simulink model "IOControls"  (R2019b)
settings: configuration reference "ConfigSet_IOControls_Reference" (kept outside this file)
model workspace (MAT data in the model file):
  SampleTime = 0.05
libraries: IOStateMachinesLib x274, SignalGeneratorsLib x1, simulink x1
(part 7 of 10)

== system IOControls/ForEachVehicle/IOControls/Non-CabControl/CircuitBreakersofEDB/SP4CB ==
  note: States:
      | Tripped
      | Set
  MCBControl : Inport  OutDataTypeStr=Bus: BD_IOControls_In_MCBControl
  Initialise : Inport  Port=2
  Bus Selector : BusSelector  OutputSignals=Value,Mode,InitVal,InternalRequest,Inhibit,TripRequest
  SP4CB-MCB : IOStateMachinesLib/MCB  InitSource=internal  InitState=InitState  OffStateValue=OffStateValue  OnStateValue=OnStateValue
      settings: SourceProductName=IO State Machines
  InputState : Outport  VectorParamsAs1DForOutWhenUnconnected=off
  MCBTripState : Outport  Port=2  VectorParamsAs1DForOutWhenUnconnected=off
  wires:
  SP4CB-MCB/2 -> MCBTripState/1
  Bus Selector/6 -> SP4CB-MCB/7  "<TripRequest>"
  MCBControl/1 -> Bus Selector/1
  Bus Selector/1 -> SP4CB-MCB/1  "<Value>"
  Bus Selector/2 -> SP4CB-MCB/2  "<Mode>"
  Bus Selector/3 -> SP4CB-MCB/3  "<InitVal>"
  Bus Selector/4 -> SP4CB-MCB/5  "<InternalRequest>"
  Bus Selector/5 -> SP4CB-MCB/6  "<Inhibit>"
  SP4CB-MCB/1 -> InputState/1
  Initialise/1 -> SP4CB-MCB/4

== system IOControls/ForEachVehicle/IOControls/Non-CabControl/CircuitBreakersofEDB/SP5CB ==
  note: States:
      | Tripped
      | Set
  MCBControl : Inport  OutDataTypeStr=Bus: BD_IOControls_In_MCBControl
  Initialise : Inport  Port=2
  Bus Selector : BusSelector  OutputSignals=Value,Mode,InitVal,InternalRequest,Inhibit,TripRequest
  SP5CB-MCB : IOStateMachinesLib/MCB  InitSource=internal  InitState=InitState  OffStateValue=OffStateValue  OnStateValue=OnStateValue
      settings: SourceProductName=IO State Machines
  InputState : Outport  VectorParamsAs1DForOutWhenUnconnected=off
  MCBTripState : Outport  Port=2  VectorParamsAs1DForOutWhenUnconnected=off
  wires:
  SP5CB-MCB/2 -> MCBTripState/1
  Bus Selector/6 -> SP5CB-MCB/7  "<TripRequest>"
  MCBControl/1 -> Bus Selector/1
  Bus Selector/1 -> SP5CB-MCB/1  "<Value>"
  Bus Selector/2 -> SP5CB-MCB/2  "<Mode>"
  Bus Selector/3 -> SP5CB-MCB/3  "<InitVal>"
  Bus Selector/4 -> SP5CB-MCB/5  "<InternalRequest>"
  Bus Selector/5 -> SP5CB-MCB/6  "<Inhibit>"
  SP5CB-MCB/1 -> InputState/1
  Initialise/1 -> SP5CB-MCB/4

== system IOControls/ForEachVehicle/IOControls/Non-CabControl/CircuitBreakersofEDB/SP6CB ==
  note: States:
      | Tripped
      | Set
  MCBControl : Inport  OutDataTypeStr=Bus: BD_IOControls_In_MCBControl
  Initialise : Inport  Port=2
  Bus Selector : BusSelector  OutputSignals=Value,Mode,InitVal,InternalRequest,Inhibit,TripRequest
  SP6CB-MCB : IOStateMachinesLib/MCB  InitSource=internal  InitState=InitState  OffStateValue=OffStateValue  OnStateValue=OnStateValue
      settings: SourceProductName=IO State Machines
  InputState : Outport  VectorParamsAs1DForOutWhenUnconnected=off
  MCBTripState : Outport  Port=2  VectorParamsAs1DForOutWhenUnconnected=off
  wires:
  SP6CB-MCB/2 -> MCBTripState/1
  Bus Selector/6 -> SP6CB-MCB/7  "<TripRequest>"
  MCBControl/1 -> Bus Selector/1
  Bus Selector/1 -> SP6CB-MCB/1  "<Value>"
  Bus Selector/2 -> SP6CB-MCB/2  "<Mode>"
  Bus Selector/3 -> SP6CB-MCB/3  "<InitVal>"
  Bus Selector/4 -> SP6CB-MCB/5  "<InternalRequest>"
  Bus Selector/5 -> SP6CB-MCB/6  "<Inhibit>"
  SP6CB-MCB/1 -> InputState/1
  Initialise/1 -> SP6CB-MCB/4

== system IOControls/ForEachVehicle/IOControls/Non-CabControl/CircuitBreakersofEDB/SPCB6 ==
  note: States:
      | Tripped
      | Set
  MCBControl : Inport  OutDataTypeStr=Bus: BD_IOControls_In_MCBControl
  Initialise : Inport  Port=2
  Bus Selector : BusSelector  OutputSignals=Value,Mode,InitVal,InternalRequest,Inhibit,TripRequest
  SPCB6-MCB : IOStateMachinesLib/MCB  InitSource=internal  InitState=InitState  OffStateValue=OffStateValue  OnStateValue=OnStateValue
      settings: SourceProductName=IO State Machines
  InputState : Outport  VectorParamsAs1DForOutWhenUnconnected=off
  MCBTripState : Outport  Port=2  VectorParamsAs1DForOutWhenUnconnected=off
  wires:
  SPCB6-MCB/2 -> MCBTripState/1
  Bus Selector/6 -> SPCB6-MCB/7  "<TripRequest>"
  MCBControl/1 -> Bus Selector/1
  Bus Selector/1 -> SPCB6-MCB/1  "<Value>"
  Bus Selector/2 -> SPCB6-MCB/2  "<Mode>"
  Bus Selector/3 -> SPCB6-MCB/3  "<InitVal>"
  Bus Selector/4 -> SPCB6-MCB/5  "<InternalRequest>"
  Bus Selector/5 -> SPCB6-MCB/6  "<Inhibit>"
  SPCB6-MCB/1 -> InputState/1
  Initialise/1 -> SPCB6-MCB/4

== system IOControls/ForEachVehicle/IOControls/Non-CabControl/CircuitBreakersofEDB/SPCB7 ==
  note: States:
      | Tripped
      | Set
  MCBControl : Inport  OutDataTypeStr=Bus: BD_IOControls_In_MCBControl
  Initialise : Inport  Port=2
  Bus Selector : BusSelector  OutputSignals=Value,Mode,InitVal,InternalRequest,Inhibit,TripRequest
  SPCB7-MCB : IOStateMachinesLib/MCB  InitSource=internal  InitState=InitState  OffStateValue=OffStateValue  OnStateValue=OnStateValue
      settings: SourceProductName=IO State Machines
  InputState : Outport  VectorParamsAs1DForOutWhenUnconnected=off
  MCBTripState : Outport  Port=2  VectorParamsAs1DForOutWhenUnconnected=off
  wires:
  SPCB7-MCB/2 -> MCBTripState/1
  Bus Selector/6 -> SPCB7-MCB/7  "<TripRequest>"
  MCBControl/1 -> Bus Selector/1
  Bus Selector/1 -> SPCB7-MCB/1  "<Value>"
  Bus Selector/2 -> SPCB7-MCB/2  "<Mode>"
  Bus Selector/3 -> SPCB7-MCB/3  "<InitVal>"
  Bus Selector/4 -> SPCB7-MCB/5  "<InternalRequest>"
  Bus Selector/5 -> SPCB7-MCB/6  "<Inhibit>"
  SPCB7-MCB/1 -> InputState/1
  Initialise/1 -> SPCB7-MCB/4

== system IOControls/ForEachVehicle/IOControls/Non-CabControl/CircuitBreakersofEDB/SPCB8 ==
  note: States:
      | Tripped
      | Set
  MCBControl : Inport  OutDataTypeStr=Bus: BD_IOControls_In_MCBControl
  Initialise : Inport  Port=2
  Bus Selector : BusSelector  OutputSignals=Value,Mode,InitVal,InternalRequest,Inhibit,TripRequest
  SPCB8-MCB : IOStateMachinesLib/MCB  InitSource=internal  InitState=InitState  OffStateValue=OffStateValue  OnStateValue=OnStateValue
      settings: SourceProductName=IO State Machines
  InputState : Outport  VectorParamsAs1DForOutWhenUnconnected=off
  MCBTripState : Outport  Port=2  VectorParamsAs1DForOutWhenUnconnected=off
  wires:
  SPCB8-MCB/2 -> MCBTripState/1
  Bus Selector/6 -> SPCB8-MCB/7  "<TripRequest>"
  MCBControl/1 -> Bus Selector/1
  Bus Selector/1 -> SPCB8-MCB/1  "<Value>"
  Bus Selector/2 -> SPCB8-MCB/2  "<Mode>"
  Bus Selector/3 -> SPCB8-MCB/3  "<InitVal>"
  Bus Selector/4 -> SPCB8-MCB/5  "<InternalRequest>"
  Bus Selector/5 -> SPCB8-MCB/6  "<Inhibit>"
  SPCB8-MCB/1 -> InputState/1
  Initialise/1 -> SPCB8-MCB/4

== system IOControls/ForEachVehicle/IOControls/Non-CabControl/CircuitBreakersofEDB/SPPB ==
  note: States:
      | Off
      | On
  InputControl : Inport  OutDataTypeStr=Bus: BD_IOControls_In_InputControl
  Initialise : Inport  Port=2
  Bus Selector : BusSelector  OutputSignals=Value,Mode,InitVal,InternalRequest,Inhibit
  SPPB-Momentary : IOStateMachinesLib/Momentary  InitSource=internal  InitState=InitState
      settings: SourceProductName=IO State Machines
  InputState : Outport  VectorParamsAs1DForOutWhenUnconnected=off
  wires:
  Initialise/1 -> SPPB-Momentary/4
  SPPB-Momentary/1 -> InputState/1
  Bus Selector/5 -> SPPB-Momentary/6  "<Inhibit>"
  Bus Selector/4 -> SPPB-Momentary/5  "<InternalRequest>"
  Bus Selector/3 -> SPPB-Momentary/3  "<InitVal>"
  Bus Selector/2 -> SPPB-Momentary/2  "<Mode>"
  Bus Selector/1 -> SPPB-Momentary/1  "<Value>"
  InputControl/1 -> Bus Selector/1

== system IOControls/ForEachVehicle/IOControls/Non-CabControl/CircuitBreakersofEDB/SPSW ==
  note: States:
      | Normal
      | Cutout
  InputControl : Inport  OutDataTypeStr=Bus: BD_IOControls_In_InputControl
  Initialise : Inport  Port=2
  Bus Selector : BusSelector  OutputSignals=Value,Mode,InitVal,InternalRequest,Inhibit
  SPSW-Toggle : IOStateMachinesLib/Toggle  InitSource=internal  InitState=InitState  OffStateValue=OffStateValue  OnStateValue=OnStateValue
      settings: SourceProductName=IO State Machines
  InputState : Outport  VectorParamsAs1DForOutWhenUnconnected=off
  wires:
  Initialise/1 -> SPSW-Toggle/4
  SPSW-Toggle/1 -> InputState/1
  Bus Selector/5 -> SPSW-Toggle/6  "<Inhibit>"
  Bus Selector/4 -> SPSW-Toggle/5  "<InternalRequest>"
  Bus Selector/3 -> SPSW-Toggle/3  "<InitVal>"
  Bus Selector/2 -> SPSW-Toggle/2  "<Mode>"
  Bus Selector/1 -> SPSW-Toggle/1  "<Value>"
  InputControl/1 -> Bus Selector/1

== system IOControls/ForEachVehicle/IOControls/Non-CabControl/CircuitBreakersofEDB/SSCB ==
  note: States:
      | Tripped
      | Set
  MCBControl : Inport  OutDataTypeStr=Bus: BD_IOControls_In_MCBControl
  Initialise : Inport  Port=2
  Bus Selector : BusSelector  OutputSignals=Value,Mode,InitVal,InternalRequest,Inhibit,TripRequest
  SSCB-MCB : IOStateMachinesLib/MCB  InitSource=internal  InitState=InitState  OffStateValue=OffStateValue  OnStateValue=OnStateValue
      settings: SourceProductName=IO State Machines
  InputState : Outport  VectorParamsAs1DForOutWhenUnconnected=off
  MCBTripState : Outport  Port=2  VectorParamsAs1DForOutWhenUnconnected=off
  wires:
  SSCB-MCB/2 -> MCBTripState/1
  Bus Selector/6 -> SSCB-MCB/7  "<TripRequest>"
  MCBControl/1 -> Bus Selector/1
  Bus Selector/1 -> SSCB-MCB/1  "<Value>"
  Bus Selector/2 -> SSCB-MCB/2  "<Mode>"
  Bus Selector/3 -> SSCB-MCB/3  "<InitVal>"
  Bus Selector/4 -> SSCB-MCB/5  "<InternalRequest>"
  Bus Selector/5 -> SSCB-MCB/6  "<Inhibit>"
  SSCB-MCB/1 -> InputState/1
  Initialise/1 -> SSCB-MCB/4

== system IOControls/ForEachVehicle/IOControls/Non-CabControl/CircuitBreakersofEDB/SSICB ==
  note: States:
      | Tripped
      | Set
  MCBControl : Inport  OutDataTypeStr=Bus: BD_IOControls_In_MCBControl
  Initialise : Inport  Port=2
  Bus Selector : BusSelector  OutputSignals=Value,Mode,InitVal,InternalRequest,Inhibit,TripRequest
  SSICB-MCB : IOStateMachinesLib/MCB  InitSource=internal  InitState=InitState  OffStateValue=OffStateValue  OnStateValue=OnStateValue
      settings: SourceProductName=IO State Machines
  InputState : Outport  VectorParamsAs1DForOutWhenUnconnected=off
  MCBTripState : Outport  Port=2  VectorParamsAs1DForOutWhenUnconnected=off
  wires:
  SSICB-MCB/2 -> MCBTripState/1
  Bus Selector/6 -> SSICB-MCB/7  "<TripRequest>"
  MCBControl/1 -> Bus Selector/1
  Bus Selector/1 -> SSICB-MCB/1  "<Value>"
  Bus Selector/2 -> SSICB-MCB/2  "<Mode>"
  Bus Selector/3 -> SSICB-MCB/3  "<InitVal>"
  Bus Selector/4 -> SSICB-MCB/5  "<InternalRequest>"
  Bus Selector/5 -> SSICB-MCB/6  "<Inhibit>"
  SSICB-MCB/1 -> InputState/1
  Initialise/1 -> SSICB-MCB/4

== system IOControls/ForEachVehicle/IOControls/Non-CabControl/CircuitBreakersofEDB/TBCCB1 ==
  note: States:
      | Tripped
      | Set
  MCBControl : Inport  OutDataTypeStr=Bus: BD_IOControls_In_MCBControl
  Initialise : Inport  Port=2
  Bus Selector : BusSelector  OutputSignals=Value,Mode,InitVal,InternalRequest,Inhibit,TripRequest
  TBCCB1-MCB : IOStateMachinesLib/MCB  InitSource=internal  InitState=InitState  OffStateValue=OffStateValue  OnStateValue=OnStateValue
      settings: SourceProductName=IO State Machines
  InputState : Outport  VectorParamsAs1DForOutWhenUnconnected=off
  MCBTripState : Outport  Port=2  VectorParamsAs1DForOutWhenUnconnected=off
  wires:
  TBCCB1-MCB/2 -> MCBTripState/1
  Bus Selector/6 -> TBCCB1-MCB/7  "<TripRequest>"
  MCBControl/1 -> Bus Selector/1
  Bus Selector/1 -> TBCCB1-MCB/1  "<Value>"
  Bus Selector/2 -> TBCCB1-MCB/2  "<Mode>"
  Bus Selector/3 -> TBCCB1-MCB/3  "<InitVal>"
  Bus Selector/4 -> TBCCB1-MCB/5  "<InternalRequest>"
  Bus Selector/5 -> TBCCB1-MCB/6  "<Inhibit>"
  TBCCB1-MCB/1 -> InputState/1
  Initialise/1 -> TBCCB1-MCB/4

== system IOControls/ForEachVehicle/IOControls/Non-CabControl/CircuitBreakersofEDB/TBCCB2 ==
  note: States:
      | Tripped
      | Set
  MCBControl : Inport  OutDataTypeStr=Bus: BD_IOControls_In_MCBControl
  Initialise : Inport  Port=2
  Bus Selector : BusSelector  OutputSignals=Value,Mode,InitVal,InternalRequest,Inhibit,TripRequest
  TBCCB2-MCB : IOStateMachinesLib/MCB  InitSource=internal  InitState=InitState  OffStateValue=OffStateValue  OnStateValue=OnStateValue
      settings: SourceProductName=IO State Machines
  InputState : Outport  VectorParamsAs1DForOutWhenUnconnected=off
  MCBTripState : Outport  Port=2  VectorParamsAs1DForOutWhenUnconnected=off
  wires:
  TBCCB2-MCB/2 -> MCBTripState/1
  Bus Selector/6 -> TBCCB2-MCB/7  "<TripRequest>"
  MCBControl/1 -> Bus Selector/1
  Bus Selector/1 -> TBCCB2-MCB/1  "<Value>"
  Bus Selector/2 -> TBCCB2-MCB/2  "<Mode>"
  Bus Selector/3 -> TBCCB2-MCB/3  "<InitVal>"
  Bus Selector/4 -> TBCCB2-MCB/5  "<InternalRequest>"
  Bus Selector/5 -> TBCCB2-MCB/6  "<Inhibit>"
  TBCCB2-MCB/1 -> InputState/1
  Initialise/1 -> TBCCB2-MCB/4

== system IOControls/ForEachVehicle/IOControls/Non-CabControl/CircuitBreakersofEDB/TBNCB ==
  note: States:
      | Tripped
      | Set
  MCBControl : Inport  OutDataTypeStr=Bus: BD_IOControls_In_MCBControl
  Initialise : Inport  Port=2
  Bus Selector : BusSelector  OutputSignals=Value,Mode,InitVal,InternalRequest,Inhibit,TripRequest
  TBNCB-MCB : IOStateMachinesLib/MCB  InitSource=internal  InitState=InitState  OffStateValue=OffStateValue  OnStateValue=OnStateValue
      settings: SourceProductName=IO State Machines
  InputState : Outport  VectorParamsAs1DForOutWhenUnconnected=off
  MCBTripState : Outport  Port=2  VectorParamsAs1DForOutWhenUnconnected=off
  wires:
  TBNCB-MCB/2 -> MCBTripState/1
  Bus Selector/6 -> TBNCB-MCB/7  "<TripRequest>"
  MCBControl/1 -> Bus Selector/1
  Bus Selector/1 -> TBNCB-MCB/1  "<Value>"
  Bus Selector/2 -> TBNCB-MCB/2  "<Mode>"
  Bus Selector/3 -> TBNCB-MCB/3  "<InitVal>"
  Bus Selector/4 -> TBNCB-MCB/5  "<InternalRequest>"
  Bus Selector/5 -> TBNCB-MCB/6  "<Inhibit>"
  TBNCB-MCB/1 -> InputState/1
  Initialise/1 -> TBNCB-MCB/4

== system IOControls/ForEachVehicle/IOControls/Non-CabControl/CircuitBreakersofEDB/TDICB ==
  note: States:
      | Tripped
      | Set
  MCBControl : Inport  OutDataTypeStr=Bus: BD_IOControls_In_MCBControl
  Initialise : Inport  Port=2
  Bus Selector : BusSelector  OutputSignals=Value,Mode,InitVal,InternalRequest,Inhibit,TripRequest
  TDICB-MCB : IOStateMachinesLib/MCB  InitSource=internal  InitState=InitState  OffStateValue=OffStateValue  OnStateValue=OnStateValue
      settings: SourceProductName=IO State Machines
  InputState : Outport  VectorParamsAs1DForOutWhenUnconnected=off
  MCBTripState : Outport  Port=2  VectorParamsAs1DForOutWhenUnconnected=off
  wires:
  TDICB-MCB/2 -> MCBTripState/1
  Bus Selector/6 -> TDICB-MCB/7  "<TripRequest>"
  MCBControl/1 -> Bus Selector/1
  Bus Selector/1 -> TDICB-MCB/1  "<Value>"
  Bus Selector/2 -> TDICB-MCB/2  "<Mode>"
  Bus Selector/3 -> TDICB-MCB/3  "<InitVal>"
  Bus Selector/4 -> TDICB-MCB/5  "<InternalRequest>"
  Bus Selector/5 -> TDICB-MCB/6  "<Inhibit>"
  TDICB-MCB/1 -> InputState/1
  Initialise/1 -> TDICB-MCB/4

== system IOControls/ForEachVehicle/IOControls/Non-CabControl/CircuitBreakersofEDB/TERCB1 ==
  note: States:
      | Tripped
      | Set
  MCBControl : Inport  OutDataTypeStr=Bus: BD_IOControls_In_MCBControl
  Initialise : Inport  Port=2
  Bus Selector : BusSelector  OutputSignals=Value,Mode,InitVal,InternalRequest,Inhibit,TripRequest
  TERCB1-MCB : IOStateMachinesLib/MCB  InitSource=internal  InitState=InitState  OffStateValue=OffStateValue  OnStateValue=OnStateValue
      settings: SourceProductName=IO State Machines
  InputState : Outport  VectorParamsAs1DForOutWhenUnconnected=off
  MCBTripState : Outport  Port=2  VectorParamsAs1DForOutWhenUnconnected=off
  wires:
  TERCB1-MCB/2 -> MCBTripState/1
  Bus Selector/6 -> TERCB1-MCB/7  "<TripRequest>"
  MCBControl/1 -> Bus Selector/1
  Bus Selector/1 -> TERCB1-MCB/1  "<Value>"
  Bus Selector/2 -> TERCB1-MCB/2  "<Mode>"
  Bus Selector/3 -> TERCB1-MCB/3  "<InitVal>"
  Bus Selector/4 -> TERCB1-MCB/5  "<InternalRequest>"
  Bus Selector/5 -> TERCB1-MCB/6  "<Inhibit>"
  TERCB1-MCB/1 -> InputState/1
  Initialise/1 -> TERCB1-MCB/4

== system IOControls/ForEachVehicle/IOControls/Non-CabControl/CircuitBreakersofEDB/TERCB2 ==
  note: States:
      | Tripped
      | Set
  MCBControl : Inport  OutDataTypeStr=Bus: BD_IOControls_In_MCBControl
  Initialise : Inport  Port=2
  Bus Selector : BusSelector  OutputSignals=Value,Mode,InitVal,InternalRequest,Inhibit,TripRequest
  TERCB2-MCB : IOStateMachinesLib/MCB  InitSource=internal  InitState=InitState  OffStateValue=OffStateValue  OnStateValue=OnStateValue
      settings: SourceProductName=IO State Machines
  InputState : Outport  VectorParamsAs1DForOutWhenUnconnected=off
  MCBTripState : Outport  Port=2  VectorParamsAs1DForOutWhenUnconnected=off
  wires:
  TERCB2-MCB/2 -> MCBTripState/1
  Bus Selector/6 -> TERCB2-MCB/7  "<TripRequest>"
  MCBControl/1 -> Bus Selector/1
  Bus Selector/1 -> TERCB2-MCB/1  "<Value>"
  Bus Selector/2 -> TERCB2-MCB/2  "<Mode>"
  Bus Selector/3 -> TERCB2-MCB/3  "<InitVal>"
  Bus Selector/4 -> TERCB2-MCB/5  "<InternalRequest>"
  Bus Selector/5 -> TERCB2-MCB/6  "<Inhibit>"
  TERCB2-MCB/1 -> InputState/1
  Initialise/1 -> TERCB2-MCB/4

== system IOControls/ForEachVehicle/IOControls/Non-CabControl/CircuitBreakersofEDB/TLLCB ==
  note: States:
      | Tripped
      | Set
  MCBControl : Inport  OutDataTypeStr=Bus: BD_IOControls_In_MCBControl
  Initialise : Inport  Port=2
  Bus Selector : BusSelector  OutputSignals=Value,Mode,InitVal,InternalRequest,Inhibit,TripRequest
  TLLCB-MCB : IOStateMachinesLib/MCB  InitSource=internal  InitState=InitState  OffStateValue=OffStateValue  OnStateValue=OnStateValue
      settings: SourceProductName=IO State Machines
  InputState : Outport  VectorParamsAs1DForOutWhenUnconnected=off
  MCBTripState : Outport  Port=2  VectorParamsAs1DForOutWhenUnconnected=off
  wires:
  TLLCB-MCB/2 -> MCBTripState/1
  Bus Selector/6 -> TLLCB-MCB/7  "<TripRequest>"
  MCBControl/1 -> Bus Selector/1
  Bus Selector/1 -> TLLCB-MCB/1  "<Value>"
  Bus Selector/2 -> TLLCB-MCB/2  "<Mode>"
  Bus Selector/3 -> TLLCB-MCB/3  "<InitVal>"
  Bus Selector/4 -> TLLCB-MCB/5  "<InternalRequest>"
  Bus Selector/5 -> TLLCB-MCB/6  "<Inhibit>"
  TLLCB-MCB/1 -> InputState/1
  Initialise/1 -> TLLCB-MCB/4

== system IOControls/ForEachVehicle/IOControls/Non-CabControl/CircuitBreakersofEDB/TLRCB ==
  note: States:
      | Tripped
      | Set
  MCBControl : Inport  OutDataTypeStr=Bus: BD_IOControls_In_MCBControl
  Initialise : Inport  Port=2
  Bus Selector : BusSelector  OutputSignals=Value,Mode,InitVal,InternalRequest,Inhibit,TripRequest
  TLRCB-MCB : IOStateMachinesLib/MCB  InitSource=internal  InitState=InitState  OffStateValue=OffStateValue  OnStateValue=OnStateValue
      settings: SourceProductName=IO State Machines
  InputState : Outport  VectorParamsAs1DForOutWhenUnconnected=off
  MCBTripState : Outport  Port=2  VectorParamsAs1DForOutWhenUnconnected=off
  wires:
  TLRCB-MCB/2 -> MCBTripState/1
  Bus Selector/6 -> TLRCB-MCB/7  "<TripRequest>"
  MCBControl/1 -> Bus Selector/1
  Bus Selector/1 -> TLRCB-MCB/1  "<Value>"
  Bus Selector/2 -> TLRCB-MCB/2  "<Mode>"
  Bus Selector/3 -> TLRCB-MCB/3  "<InitVal>"
  Bus Selector/4 -> TLRCB-MCB/5  "<InternalRequest>"
  Bus Selector/5 -> TLRCB-MCB/6  "<Inhibit>"
  TLRCB-MCB/1 -> InputState/1
  Initialise/1 -> TLRCB-MCB/4

== system IOControls/ForEachVehicle/IOControls/Non-CabControl/CircuitBreakersofEDB/TRIVCB ==
  note: States:
      | Tripped
      | Set
  MCBControl : Inport  OutDataTypeStr=Bus: BD_IOControls_In_MCBControl
  Initialise : Inport  Port=2
  Bus Selector : BusSelector  OutputSignals=Value,Mode,InitVal,InternalRequest,Inhibit,TripRequest
  TRIVCB-MCB : IOStateMachinesLib/MCB  InitSource=internal  InitState=InitState  OffStateValue=OffStateValue  OnStateValue=OnStateValue
      settings: SourceProductName=IO State Machines
  InputState : Outport  VectorParamsAs1DForOutWhenUnconnected=off
  MCBTripState : Outport  Port=2  VectorParamsAs1DForOutWhenUnconnected=off
  wires:
  TRIVCB-MCB/2 -> MCBTripState/1
  Bus Selector/6 -> TRIVCB-MCB/7  "<TripRequest>"
  MCBControl/1 -> Bus Selector/1
  Bus Selector/1 -> TRIVCB-MCB/1  "<Value>"
  Bus Selector/2 -> TRIVCB-MCB/2  "<Mode>"
  Bus Selector/3 -> TRIVCB-MCB/3  "<InitVal>"
  Bus Selector/4 -> TRIVCB-MCB/5  "<InternalRequest>"
  Bus Selector/5 -> TRIVCB-MCB/6  "<Inhibit>"
  TRIVCB-MCB/1 -> InputState/1
  Initialise/1 -> TRIVCB-MCB/4

== system IOControls/ForEachVehicle/IOControls/Non-CabControl/CircuitBreakersofEDB/TVDUCB ==
  note: States:
      | Tripped
      | Set
  MCBControl : Inport  OutDataTypeStr=Bus: BD_IOControls_In_MCBControl
  Initialise : Inport  Port=2
  Bus Selector : BusSelector  OutputSignals=Value,Mode,InitVal,InternalRequest,Inhibit,TripRequest
  TVDUCB-MCB : IOStateMachinesLib/MCB  InitSource=internal  InitState=InitState  OffStateValue=OffStateValue  OnStateValue=OnStateValue
      settings: SourceProductName=IO State Machines
  InputState : Outport  VectorParamsAs1DForOutWhenUnconnected=off
  MCBTripState : Outport  Port=2  VectorParamsAs1DForOutWhenUnconnected=off
  wires:
  TVDUCB-MCB/2 -> MCBTripState/1
  Bus Selector/6 -> TVDUCB-MCB/7  "<TripRequest>"
  MCBControl/1 -> Bus Selector/1
  Bus Selector/1 -> TVDUCB-MCB/1  "<Value>"
  Bus Selector/2 -> TVDUCB-MCB/2  "<Mode>"
  Bus Selector/3 -> TVDUCB-MCB/3  "<InitVal>"
  Bus Selector/4 -> TVDUCB-MCB/5  "<InternalRequest>"
  Bus Selector/5 -> TVDUCB-MCB/6  "<Inhibit>"
  TVDUCB-MCB/1 -> InputState/1
  Initialise/1 -> TVDUCB-MCB/4

== system IOControls/ForEachVehicle/IOControls/Non-CabControl/CircuitBreakersofEDB/TWVCB ==
  note: States:
      | Tripped
      | Set
  MCBControl : Inport  OutDataTypeStr=Bus: BD_IOControls_In_MCBControl
  Initialise : Inport  Port=2
  Bus Selector : BusSelector  OutputSignals=Value,Mode,InitVal,InternalRequest,Inhibit,TripRequest
  TWVCB-MCB : IOStateMachinesLib/MCB  InitSource=internal  InitState=InitState  OffStateValue=OffStateValue  OnStateValue=OnStateValue
      settings: SourceProductName=IO State Machines
  InputState : Outport  VectorParamsAs1DForOutWhenUnconnected=off
  MCBTripState : Outport  Port=2  VectorParamsAs1DForOutWhenUnconnected=off
  wires:
  TWVCB-MCB/2 -> MCBTripState/1
  Bus Selector/6 -> TWVCB-MCB/7  "<TripRequest>"
  MCBControl/1 -> Bus Selector/1
  Bus Selector/1 -> TWVCB-MCB/1  "<Value>"
  Bus Selector/2 -> TWVCB-MCB/2  "<Mode>"
  Bus Selector/3 -> TWVCB-MCB/3  "<InitVal>"
  Bus Selector/4 -> TWVCB-MCB/5  "<InternalRequest>"
  Bus Selector/5 -> TWVCB-MCB/6  "<Inhibit>"
  TWVCB-MCB/1 -> InputState/1
  Initialise/1 -> TWVCB-MCB/4

== system IOControls/ForEachVehicle/IOControls/Non-CabControl/CircuitBreakersofEDB/VCBCB ==
  note: States:
      | Tripped
      | Set
  MCBControl : Inport  OutDataTypeStr=Bus: BD_IOControls_In_MCBControl
  Initialise : Inport  Port=2
  Bus Selector : BusSelector  OutputSignals=Value,Mode,InitVal,InternalRequest,Inhibit,TripRequest
  VCBCB-MCB : IOStateMachinesLib/MCB  InitSource=internal  InitState=InitState  OffStateValue=OffStateValue  OnStateValue=OnStateValue
      settings: SourceProductName=IO State Machines
  InputState : Outport  VectorParamsAs1DForOutWhenUnconnected=off
  MCBTripState : Outport  Port=2  VectorParamsAs1DForOutWhenUnconnected=off
  wires:
  VCBCB-MCB/2 -> MCBTripState/1
  Bus Selector/6 -> VCBCB-MCB/7  "<TripRequest>"
  MCBControl/1 -> Bus Selector/1
  Bus Selector/1 -> VCBCB-MCB/1  "<Value>"
  Bus Selector/2 -> VCBCB-MCB/2  "<Mode>"
  Bus Selector/3 -> VCBCB-MCB/3  "<InitVal>"
  Bus Selector/4 -> VCBCB-MCB/5  "<InternalRequest>"
  Bus Selector/5 -> VCBCB-MCB/6  "<Inhibit>"
  VCBCB-MCB/1 -> InputState/1
  Initialise/1 -> VCBCB-MCB/4

== system IOControls/ForEachVehicle/IOControls/Non-CabControl/CircuitBreakersofEDB/VCBCCB ==
  note: States:
      | Tripped
      | Set
  MCBControl : Inport  OutDataTypeStr=Bus: BD_IOControls_In_MCBControl
  Initialise : Inport  Port=2
  Bus Selector : BusSelector  OutputSignals=Value,Mode,InitVal,InternalRequest,Inhibit,TripRequest
  VCBCCB-MCB : IOStateMachinesLib/MCB  InitSource=internal  InitState=InitState  OffStateValue=OffStateValue  OnStateValue=OnStateValue
      settings: SourceProductName=IO State Machines
  InputState : Outport  VectorParamsAs1DForOutWhenUnconnected=off
  MCBTripState : Outport  Port=2  VectorParamsAs1DForOutWhenUnconnected=off
  wires:
  VCBCCB-MCB/2 -> MCBTripState/1
  Bus Selector/6 -> VCBCCB-MCB/7  "<TripRequest>"
  MCBControl/1 -> Bus Selector/1
  Bus Selector/1 -> VCBCCB-MCB/1  "<Value>"
  Bus Selector/2 -> VCBCCB-MCB/2  "<Mode>"
  Bus Selector/3 -> VCBCCB-MCB/3  "<InitVal>"
  Bus Selector/4 -> VCBCCB-MCB/5  "<InternalRequest>"
  Bus Selector/5 -> VCBCCB-MCB/6  "<Inhibit>"
  VCBCCB-MCB/1 -> InputState/1
  Initialise/1 -> VCBCCB-MCB/4

== system IOControls/ForEachVehicle/IOControls/Non-CabControl/CircuitBreakersofEDB/VCCBOrUCCB ==
  note: States:
      | Tripped
      | Set
  MCBControl : Inport  OutDataTypeStr=Bus: BD_IOControls_In_MCBControl
  Initialise : Inport  Port=2
  Bus Selector : BusSelector  OutputSignals=Value,Mode,InitVal,InternalRequest,Inhibit,TripRequest
  VCCBOrUCCB-MCB : IOStateMachinesLib/MCB  InitSource=internal  InitState=InitState  OffStateValue=OffStateValue  OnStateValue=OnStateValue
      settings: SourceProductName=IO State Machines
  InputState : Outport  VectorParamsAs1DForOutWhenUnconnected=off
  MCBTripState : Outport  Port=2  VectorParamsAs1DForOutWhenUnconnected=off
  wires:
  VCCBOrUCCB-MCB/2 -> MCBTripState/1
  Bus Selector/6 -> VCCBOrUCCB-MCB/7  "<TripRequest>"
  MCBControl/1 -> Bus Selector/1
  Bus Selector/1 -> VCCBOrUCCB-MCB/1  "<Value>"
  Bus Selector/2 -> VCCBOrUCCB-MCB/2  "<Mode>"
  Bus Selector/3 -> VCCBOrUCCB-MCB/3  "<InitVal>"
  Bus Selector/4 -> VCCBOrUCCB-MCB/5  "<InternalRequest>"
  Bus Selector/5 -> VCCBOrUCCB-MCB/6  "<Inhibit>"
  VCCBOrUCCB-MCB/1 -> InputState/1
  Initialise/1 -> VCCBOrUCCB-MCB/4

== system IOControls/ForEachVehicle/IOControls/Non-CabControl/CircuitBreakersofEDB/VIO1CB ==
  note: States:
      | Tripped
      | Set
  MCBControl : Inport  OutDataTypeStr=Bus: BD_IOControls_In_MCBControl
  Initialise : Inport  Port=2
  Bus Selector : BusSelector  OutputSignals=Value,Mode,InitVal,InternalRequest,Inhibit,TripRequest
  VIO1CB-MCB : IOStateMachinesLib/MCB  InitSource=internal  InitState=InitState  OffStateValue=OffStateValue  OnStateValue=OnStateValue
      settings: SourceProductName=IO State Machines
  InputState : Outport  VectorParamsAs1DForOutWhenUnconnected=off
  MCBTripState : Outport  Port=2  VectorParamsAs1DForOutWhenUnconnected=off
  wires:
  VIO1CB-MCB/2 -> MCBTripState/1
  Bus Selector/6 -> VIO1CB-MCB/7  "<TripRequest>"
  MCBControl/1 -> Bus Selector/1
  Bus Selector/1 -> VIO1CB-MCB/1  "<Value>"
  Bus Selector/2 -> VIO1CB-MCB/2  "<Mode>"
  Bus Selector/3 -> VIO1CB-MCB/3  "<InitVal>"
  Bus Selector/4 -> VIO1CB-MCB/5  "<InternalRequest>"
  Bus Selector/5 -> VIO1CB-MCB/6  "<Inhibit>"
  VIO1CB-MCB/1 -> InputState/1
  Initialise/1 -> VIO1CB-MCB/4

== system IOControls/ForEachVehicle/IOControls/Non-CabControl/CircuitBreakersofEDB/VIO2CB ==
  note: States:
      | Tripped
      | Set
  MCBControl : Inport  OutDataTypeStr=Bus: BD_IOControls_In_MCBControl
  Initialise : Inport  Port=2
  Bus Selector : BusSelector  OutputSignals=Value,Mode,InitVal,InternalRequest,Inhibit,TripRequest
  VIO2CB-MCB : IOStateMachinesLib/MCB  InitSource=internal  InitState=InitState  OffStateValue=OffStateValue  OnStateValue=OnStateValue
      settings: SourceProductName=IO State Machines
  InputState : Outport  VectorParamsAs1DForOutWhenUnconnected=off
  MCBTripState : Outport  Port=2  VectorParamsAs1DForOutWhenUnconnected=off
  wires:
  VIO2CB-MCB/2 -> MCBTripState/1
  Bus Selector/6 -> VIO2CB-MCB/7  "<TripRequest>"
  MCBControl/1 -> Bus Selector/1
  Bus Selector/1 -> VIO2CB-MCB/1  "<Value>"
  Bus Selector/2 -> VIO2CB-MCB/2  "<Mode>"
  Bus Selector/3 -> VIO2CB-MCB/3  "<InitVal>"
  Bus Selector/4 -> VIO2CB-MCB/5  "<InternalRequest>"
  Bus Selector/5 -> VIO2CB-MCB/6  "<Inhibit>"
  VIO2CB-MCB/1 -> InputState/1
  Initialise/1 -> VIO2CB-MCB/4

== system IOControls/ForEachVehicle/IOControls/Non-CabControl/CircuitBreakersofEDB/WFLCB ==
  note: States:
      | Tripped
      | Set
  MCBControl : Inport  OutDataTypeStr=Bus: BD_IOControls_In_MCBControl
  Initialise : Inport  Port=2
  Bus Selector : BusSelector  OutputSignals=Value,Mode,InitVal,InternalRequest,Inhibit,TripRequest
  WFLCB-MCB : IOStateMachinesLib/MCB  InitSource=internal  InitState=InitState  OffStateValue=OffStateValue  OnStateValue=OnStateValue
      settings: SourceProductName=IO State Machines
  InputState : Outport  VectorParamsAs1DForOutWhenUnconnected=off
  MCBTripState : Outport  Port=2  VectorParamsAs1DForOutWhenUnconnected=off
  wires:
  WFLCB-MCB/2 -> MCBTripState/1
  Bus Selector/6 -> WFLCB-MCB/7  "<TripRequest>"
  MCBControl/1 -> Bus Selector/1
  Bus Selector/1 -> WFLCB-MCB/1  "<Value>"
  Bus Selector/2 -> WFLCB-MCB/2  "<Mode>"
  Bus Selector/3 -> WFLCB-MCB/3  "<InitVal>"
  Bus Selector/4 -> WFLCB-MCB/5  "<InternalRequest>"
  Bus Selector/5 -> WFLCB-MCB/6  "<Inhibit>"
  WFLCB-MCB/1 -> InputState/1
  Initialise/1 -> WFLCB-MCB/4

== system IOControls/ForEachVehicle/IOControls/Non-CabControl/CircuitBreakersofEDB/WIFICB ==
  note: States:
      | Tripped
      | Set
  MCBControl : Inport  OutDataTypeStr=Bus: BD_IOControls_In_MCBControl
  Initialise : Inport  Port=2
  Bus Selector : BusSelector  OutputSignals=Value,Mode,InitVal,InternalRequest,Inhibit,TripRequest
  WIFICB-MCB : IOStateMachinesLib/MCB  InitSource=internal  InitState=InitState  OffStateValue=OffStateValue  OnStateValue=OnStateValue
      settings: SourceProductName=IO State Machines
  InputState : Outport  VectorParamsAs1DForOutWhenUnconnected=off
  MCBTripState : Outport  Port=2  VectorParamsAs1DForOutWhenUnconnected=off
  wires:
  WIFICB-MCB/2 -> MCBTripState/1
  Bus Selector/6 -> WIFICB-MCB/7  "<TripRequest>"
  MCBControl/1 -> Bus Selector/1
  Bus Selector/1 -> WIFICB-MCB/1  "<Value>"
  Bus Selector/2 -> WIFICB-MCB/2  "<Mode>"
  Bus Selector/3 -> WIFICB-MCB/3  "<InitVal>"
  Bus Selector/4 -> WIFICB-MCB/5  "<InternalRequest>"
  Bus Selector/5 -> WIFICB-MCB/6  "<Inhibit>"
  WIFICB-MCB/1 -> InputState/1
  Initialise/1 -> WIFICB-MCB/4

== system IOControls/ForEachVehicle/IOControls/Non-CabControl/CircuitBreakersofEDB/WWCB ==
  note: States:
      | Tripped
      | Set
  MCBControl : Inport  OutDataTypeStr=Bus: BD_IOControls_In_MCBControl
  Initialise : Inport  Port=2
  Bus Selector : BusSelector  OutputSignals=Value,Mode,InitVal,InternalRequest,Inhibit,TripRequest
  WWCB-MCB : IOStateMachinesLib/MCB  InitSource=internal  InitState=InitState  OffStateValue=OffStateValue  OnStateValue=OnStateValue
      settings: SourceProductName=IO State Machines
  InputState : Outport  VectorParamsAs1DForOutWhenUnconnected=off
  MCBTripState : Outport  Port=2  VectorParamsAs1DForOutWhenUnconnected=off
  wires:
  WWCB-MCB/2 -> MCBTripState/1
  Bus Selector/6 -> WWCB-MCB/7  "<TripRequest>"
  MCBControl/1 -> Bus Selector/1
  Bus Selector/1 -> WWCB-MCB/1  "<Value>"
  Bus Selector/2 -> WWCB-MCB/2  "<Mode>"
  Bus Selector/3 -> WWCB-MCB/3  "<InitVal>"
  Bus Selector/4 -> WWCB-MCB/5  "<InternalRequest>"
  Bus Selector/5 -> WWCB-MCB/6  "<Inhibit>"
  WWCB-MCB/1 -> InputState/1
  Initialise/1 -> WWCB-MCB/4

== system IOControls/ForEachVehicle/IOControls/Non-CabControl/CircuitBreakersofEDB/ZVBACB ==
  note: States:
      | Tripped
      | Set
  MCBControl : Inport  OutDataTypeStr=Bus: BD_IOControls_In_MCBControl
  Initialise : Inport  Port=2
  Bus Selector : BusSelector  OutputSignals=Value,Mode,InitVal,InternalRequest,Inhibit,TripRequest
  ZVBACB-MCB : IOStateMachinesLib/MCB  InitSource=internal  InitState=InitState  OffStateValue=OffStateValue  OnStateValue=OnStateValue
      settings: SourceProductName=IO State Machines
  InputState : Outport  VectorParamsAs1DForOutWhenUnconnected=off
  MCBTripState : Outport  Port=2  VectorParamsAs1DForOutWhenUnconnected=off
  wires:
  ZVBACB-MCB/2 -> MCBTripState/1
  Bus Selector/6 -> ZVBACB-MCB/7  "<TripRequest>"
  MCBControl/1 -> Bus Selector/1
  Bus Selector/1 -> ZVBACB-MCB/1  "<Value>"
  Bus Selector/2 -> ZVBACB-MCB/2  "<Mode>"
  Bus Selector/3 -> ZVBACB-MCB/3  "<InitVal>"
  Bus Selector/4 -> ZVBACB-MCB/5  "<InternalRequest>"
  Bus Selector/5 -> ZVBACB-MCB/6  "<Inhibit>"
  ZVBACB-MCB/1 -> InputState/1
  Initialise/1 -> ZVBACB-MCB/4

== system IOControls/ForEachVehicle/IOControls/Non-CabControl/EDBPanel/ORDPlunger ==
  note: States:
      | Normal
      | Pulled
  InputControl : Inport  OutDataTypeStr=Bus: BD_IOControls_In_InputControl
  Initialise : Inport  Port=2
  Bus Selector : BusSelector  OutputSignals=Value,Mode,InitVal,InternalRequest,Inhibit
  ORDPlunger-Toggle : IOStateMachinesLib/Toggle  InitSource=internal  InitState=InitState  OffStateValue=OffStateValue  OnStateValue=OnStateValue
      settings: SourceProductName=IO State Machines
  InputState : Outport  VectorParamsAs1DForOutWhenUnconnected=off
  wires:
  Initialise/1 -> ORDPlunger-Toggle/4
  ORDPlunger-Toggle/1 -> InputState/1
  Bus Selector/5 -> ORDPlunger-Toggle/6  "<Inhibit>"
  Bus Selector/4 -> ORDPlunger-Toggle/5  "<InternalRequest>"
  Bus Selector/3 -> ORDPlunger-Toggle/3  "<InitVal>"
  Bus Selector/2 -> ORDPlunger-Toggle/2  "<Mode>"
  Bus Selector/1 -> ORDPlunger-Toggle/1  "<Value>"
  InputControl/1 -> Bus Selector/1

== system IOControls/ForEachVehicle/IOControls/Non-CabControl/EDBPanel/PantographIsolationCock ==
  note: States:
      | Isolated
      | Normal
  InputControl : Inport  OutDataTypeStr=Bus: BD_IOControls_In_InputControl
  Initialise : Inport  Port=2
  Bus Selector : BusSelector  OutputSignals=Value,Mode,InitVal,InternalRequest,Inhibit
  PantographIsolationCock-Toggle : IOStateMachinesLib/Toggle  InitSource=internal  InitState=InitState  OffStateValue=OffStateValue  OnStateValue=OnStateValue
      settings: SourceProductName=IO State Machines
  InputState : Outport  VectorParamsAs1DForOutWhenUnconnected=off
  wires:
  Initialise/1 -> PantographIsolationCock-Toggle/4
  PantographIsolationCock-Toggle/1 -> InputState/1
  Bus Selector/5 -> PantographIsolationCock-Toggle/6  "<Inhibit>"
  Bus Selector/4 -> PantographIsolationCock-Toggle/5  "<InternalRequest>"
  Bus Selector/3 -> PantographIsolationCock-Toggle/3  "<InitVal>"
  Bus Selector/2 -> PantographIsolationCock-Toggle/2  "<Mode>"
  Bus Selector/1 -> PantographIsolationCock-Toggle/1  "<Value>"
  InputControl/1 -> Bus Selector/1

== system IOControls/ForEachVehicle/IOControls/Non-CabControl/EDBPanel/VCBIsolationCock ==
  note: States:
      | Isolated
      | Normal
  InputControl : Inport  OutDataTypeStr=Bus: BD_IOControls_In_InputControl
  Initialise : Inport  Port=2
  Bus Selector : BusSelector  OutputSignals=Value,Mode,InitVal,InternalRequest,Inhibit
  VCBIsolationCock-Toggle : IOStateMachinesLib/Toggle  InitSource=internal  InitState=InitState  OffStateValue=OffStateValue  OnStateValue=OnStateValue
      settings: SourceProductName=IO State Machines
  InputState : Outport  VectorParamsAs1DForOutWhenUnconnected=off
  wires:
  Initialise/1 -> VCBIsolationCock-Toggle/4
  VCBIsolationCock-Toggle/1 -> InputState/1
  Bus Selector/5 -> VCBIsolationCock-Toggle/6  "<Inhibit>"
  Bus Selector/4 -> VCBIsolationCock-Toggle/5  "<InternalRequest>"
  Bus Selector/3 -> VCBIsolationCock-Toggle/3  "<InitVal>"
  Bus Selector/2 -> VCBIsolationCock-Toggle/2  "<Mode>"
  Bus Selector/1 -> VCBIsolationCock-Toggle/1  "<Value>"
  InputControl/1 -> Bus Selector/1

== system IOControls/ForEachVehicle/IOControls/Non-CabControl/ExteriorDoorControls/LeftDoorEAD ==
  note: States:
      | Reset
      | Unlock
  InputControl : Inport  OutDataTypeStr=Bus: BD_IOControls_In_InputControl
  Initialise : Inport  Port=2
  Bus Selector : BusSelector  OutputSignals=Value,Mode,InitVal,InternalRequest,Inhibit
  LeftDoorEAD-Momentary : IOStateMachinesLib/Momentary  InitSource=internal  InitState=InitState
      settings: SourceProductName=IO State Machines
  InputState : Outport  VectorParamsAs1DForOutWhenUnconnected=off
  wires:
  Initialise/1 -> LeftDoorEAD-Momentary/4
  LeftDoorEAD-Momentary/1 -> InputState/1
  Bus Selector/5 -> LeftDoorEAD-Momentary/6  "<Inhibit>"
  Bus Selector/4 -> LeftDoorEAD-Momentary/5  "<InternalRequest>"
  Bus Selector/3 -> LeftDoorEAD-Momentary/3  "<InitVal>"
  Bus Selector/2 -> LeftDoorEAD-Momentary/2  "<Mode>"
  Bus Selector/1 -> LeftDoorEAD-Momentary/1  "<Value>"
  InputControl/1 -> Bus Selector/1

== system IOControls/ForEachVehicle/IOControls/Non-CabControl/ExteriorDoorControls/LeftDoorEADCover ==
  note: States:
      | Closed
      | Open
  InputControl : Inport  OutDataTypeStr=Bus: BD_IOControls_In_InputControl
  Initialise : Inport  Port=2
  Bus Selector : BusSelector  OutputSignals=Value,Mode,InitVal,InternalRequest,Inhibit
  LeftDoorEADCover-Toggle : IOStateMachinesLib/Toggle  InitSource=internal  InitState=InitState  OffStateValue=OffStateValue  OnStateValue=OnStateValue
      settings: SourceProductName=IO State Machines
  InputState : Outport  VectorParamsAs1DForOutWhenUnconnected=off
  wires:
  Initialise/1 -> LeftDoorEADCover-Toggle/4
  LeftDoorEADCover-Toggle/1 -> InputState/1
  Bus Selector/5 -> LeftDoorEADCover-Toggle/6  "<Inhibit>"
  Bus Selector/4 -> LeftDoorEADCover-Toggle/5  "<InternalRequest>"
  Bus Selector/3 -> LeftDoorEADCover-Toggle/3  "<InitVal>"
  Bus Selector/2 -> LeftDoorEADCover-Toggle/2  "<Mode>"
  Bus Selector/1 -> LeftDoorEADCover-Toggle/1  "<Value>"
  InputControl/1 -> Bus Selector/1

== system IOControls/ForEachVehicle/IOControls/Non-CabControl/ExteriorDoorControls/RightDoorEAD ==
  note: States:
      | Reset
      | Unlock
  InputControl : Inport  OutDataTypeStr=Bus: BD_IOControls_In_InputControl
  Initialise : Inport  Port=2
  Bus Selector : BusSelector  OutputSignals=Value,Mode,InitVal,InternalRequest,Inhibit
  RightDoorEAD-Momentary : IOStateMachinesLib/Momentary  InitSource=internal  InitState=InitState
      settings: SourceProductName=IO State Machines
  InputState : Outport  VectorParamsAs1DForOutWhenUnconnected=off
  wires:
  Initialise/1 -> RightDoorEAD-Momentary/4
  RightDoorEAD-Momentary/1 -> InputState/1
  Bus Selector/5 -> RightDoorEAD-Momentary/6  "<Inhibit>"
  Bus Selector/4 -> RightDoorEAD-Momentary/5  "<InternalRequest>"
  Bus Selector/3 -> RightDoorEAD-Momentary/3  "<InitVal>"
  Bus Selector/2 -> RightDoorEAD-Momentary/2  "<Mode>"
  Bus Selector/1 -> RightDoorEAD-Momentary/1  "<Value>"
  InputControl/1 -> Bus Selector/1

== system IOControls/ForEachVehicle/IOControls/Non-CabControl/ExteriorDoorControls/RightDoorEADCover ==
  note: States:
      | Closed
      | Open
  InputControl : Inport  OutDataTypeStr=Bus: BD_IOControls_In_InputControl
  Initialise : Inport  Port=2
  Bus Selector : BusSelector  OutputSignals=Value,Mode,InitVal,InternalRequest,Inhibit
  RightDoorEADCover-Toggle : IOStateMachinesLib/Toggle  InitSource=internal  InitState=InitState  OffStateValue=OffStateValue  OnStateValue=OnStateValue
      settings: SourceProductName=IO State Machines
  InputState : Outport  VectorParamsAs1DForOutWhenUnconnected=off
  wires:
  Initialise/1 -> RightDoorEADCover-Toggle/4
  RightDoorEADCover-Toggle/1 -> InputState/1
  Bus Selector/5 -> RightDoorEADCover-Toggle/6  "<Inhibit>"
  Bus Selector/4 -> RightDoorEADCover-Toggle/5  "<InternalRequest>"
  Bus Selector/3 -> RightDoorEADCover-Toggle/3  "<InitVal>"
  Bus Selector/2 -> RightDoorEADCover-Toggle/2  "<Mode>"
  Bus Selector/1 -> RightDoorEADCover-Toggle/1  "<Value>"
  InputControl/1 -> Bus Selector/1

== system IOControls/ForEachVehicle/IOControls/Non-CabControl/InteriorDoorControls/LeftDoor1Coving ==
  note: States:
      | Closed
      | Open
  InputControl : Inport  OutDataTypeStr=Bus: BD_IOControls_In_InputControl
  Initialise : Inport  Port=2
  Bus Selector : BusSelector  OutputSignals=Value,Mode,InitVal,InternalRequest,Inhibit
  LeftDoor1Coving-Toggle : IOStateMachinesLib/Toggle  InitSource=internal  InitState=InitState  OffStateValue=OffStateValue  OnStateValue=OnStateValue
      settings: SourceProductName=IO State Machines
  InputState : Outport  VectorParamsAs1DForOutWhenUnconnected=off
  wires:
  Initialise/1 -> LeftDoor1Coving-Toggle/4
  LeftDoor1Coving-Toggle/1 -> InputState/1
  Bus Selector/5 -> LeftDoor1Coving-Toggle/6  "<Inhibit>"
  Bus Selector/4 -> LeftDoor1Coving-Toggle/5  "<InternalRequest>"
  Bus Selector/3 -> LeftDoor1Coving-Toggle/3  "<InitVal>"
  Bus Selector/2 -> LeftDoor1Coving-Toggle/2  "<Mode>"
  Bus Selector/1 -> LeftDoor1Coving-Toggle/1  "<Value>"
  InputControl/1 -> Bus Selector/1

== system IOControls/ForEachVehicle/IOControls/Non-CabControl/InteriorDoorControls/LeftDoor1DCUCB ==
  note: States:
      | Tripped
      | Set
  MCBControl : Inport  OutDataTypeStr=Bus: BD_IOControls_In_MCBControl
  Initialise : Inport  Port=2
  Bus Selector : BusSelector  OutputSignals=Value,Mode,InitVal,InternalRequest,Inhibit,TripRequest
  LeftDoor1DCUCB-MCB : IOStateMachinesLib/MCB  InitSource=internal  InitState=InitState  OffStateValue=OffStateValue  OnStateValue=OnStateValue
      settings: SourceProductName=IO State Machines
  InputState : Outport  VectorParamsAs1DForOutWhenUnconnected=off
  MCBTripState : Outport  Port=2  VectorParamsAs1DForOutWhenUnconnected=off
  wires:
  LeftDoor1DCUCB-MCB/2 -> MCBTripState/1
  Bus Selector/6 -> LeftDoor1DCUCB-MCB/7  "<TripRequest>"
  MCBControl/1 -> Bus Selector/1
  Bus Selector/1 -> LeftDoor1DCUCB-MCB/1  "<Value>"
  Bus Selector/2 -> LeftDoor1DCUCB-MCB/2  "<Mode>"
  Bus Selector/3 -> LeftDoor1DCUCB-MCB/3  "<InitVal>"
  Bus Selector/4 -> LeftDoor1DCUCB-MCB/5  "<InternalRequest>"
  Bus Selector/5 -> LeftDoor1DCUCB-MCB/6  "<Inhibit>"
  LeftDoor1DCUCB-MCB/1 -> InputState/1
  Initialise/1 -> LeftDoor1DCUCB-MCB/4

== system IOControls/ForEachVehicle/IOControls/Non-CabControl/InteriorDoorControls/LeftDoor1EED ==
  note: States:
      | Reset
      | Operated
  InputControl : Inport  OutDataTypeStr=Bus: BD_IOControls_In_InputControl
  Initialise : Inport  Port=2
  Bus Selector : BusSelector  OutputSignals=Value,Mode,InitVal,InternalRequest,Inhibit
  LeftDoor1EED-Momentary : IOStateMachinesLib/Momentary  InitSource=internal  InitState=InitState
      settings: SourceProductName=IO State Machines
  InputState : Outport  VectorParamsAs1DForOutWhenUnconnected=off
  wires:
  Initialise/1 -> LeftDoor1EED-Momentary/4
  LeftDoor1EED-Momentary/1 -> InputState/1
  Bus Selector/5 -> LeftDoor1EED-Momentary/6  "<Inhibit>"
  Bus Selector/4 -> LeftDoor1EED-Momentary/5  "<InternalRequest>"
  Bus Selector/3 -> LeftDoor1EED-Momentary/3  "<InitVal>"
  Bus Selector/2 -> LeftDoor1EED-Momentary/2  "<Mode>"
  Bus Selector/1 -> LeftDoor1EED-Momentary/1  "<Value>"
  InputControl/1 -> Bus Selector/1

== system IOControls/ForEachVehicle/IOControls/Non-CabControl/InteriorDoorControls/LeftDoor1Lockout ==
  note: States:
      | Unlocked
      | Locked
  InputControl : Inport  OutDataTypeStr=Bus: BD_IOControls_In_InputControl
  Initialise : Inport  Port=2
  Bus Selector : BusSelector  OutputSignals=Value,Mode,InitVal,InternalRequest,Inhibit
  LeftDoor1Lockout-Toggle : IOStateMachinesLib/Toggle  InitSource=internal  InitState=InitState  OffStateValue=OffStateValue  OnStateValue=OnStateValue
      settings: SourceProductName=IO State Machines
  InputState : Outport  VectorParamsAs1DForOutWhenUnconnected=off
  wires:
  Initialise/1 -> LeftDoor1Lockout-Toggle/4
  LeftDoor1Lockout-Toggle/1 -> InputState/1
  Bus Selector/5 -> LeftDoor1Lockout-Toggle/6  "<Inhibit>"
  Bus Selector/4 -> LeftDoor1Lockout-Toggle/5  "<InternalRequest>"
  Bus Selector/3 -> LeftDoor1Lockout-Toggle/3  "<InitVal>"
  Bus Selector/2 -> LeftDoor1Lockout-Toggle/2  "<Mode>"
  Bus Selector/1 -> LeftDoor1Lockout-Toggle/1  "<Value>"
  InputControl/1 -> Bus Selector/1

== system IOControls/ForEachVehicle/IOControls/Non-CabControl/InteriorDoorControls/LeftDoor1ManualClose ==
  note: States:
      | Close
      | Open
  InputControl : Inport  OutDataTypeStr=Bus: BD_IOControls_In_InputControl
  Initialise : Inport  Port=2
  Bus Selector : BusSelector  OutputSignals=Value,Mode,InitVal,InternalRequest,Inhibit
  LeftDoor1ManualClose-Momentary : IOStateMachinesLib/Momentary  InitSource=internal  InitState=InitState
      settings: SourceProductName=IO State Machines
  InputState : Outport  VectorParamsAs1DForOutWhenUnconnected=off
  wires:
  Initialise/1 -> LeftDoor1ManualClose-Momentary/4
  LeftDoor1ManualClose-Momentary/1 -> InputState/1
  Bus Selector/5 -> LeftDoor1ManualClose-Momentary/6  "<Inhibit>"
  Bus Selector/4 -> LeftDoor1ManualClose-Momentary/5  "<InternalRequest>"
  Bus Selector/3 -> LeftDoor1ManualClose-Momentary/3  "<InitVal>"
  Bus Selector/2 -> LeftDoor1ManualClose-Momentary/2  "<Mode>"
  Bus Selector/1 -> LeftDoor1ManualClose-Momentary/1  "<Value>"
  InputControl/1 -> Bus Selector/1

== system IOControls/ForEachVehicle/IOControls/Non-CabControl/InteriorDoorControls/LeftDoor1ManualOpen ==
  note: States:
      | Close
      | Open
  InputControl : Inport  OutDataTypeStr=Bus: BD_IOControls_In_InputControl
  Initialise : Inport  Port=2
  Bus Selector : BusSelector  OutputSignals=Value,Mode,InitVal,InternalRequest,Inhibit
  LeftDoor1ManualOpen-Momentary : IOStateMachinesLib/Momentary  InitSource=internal  InitState=InitState
      settings: SourceProductName=IO State Machines
  InputState : Outport  VectorParamsAs1DForOutWhenUnconnected=off
  wires:
  Initialise/1 -> LeftDoor1ManualOpen-Momentary/4
  LeftDoor1ManualOpen-Momentary/1 -> InputState/1
  Bus Selector/5 -> LeftDoor1ManualOpen-Momentary/6  "<Inhibit>"
  Bus Selector/4 -> LeftDoor1ManualOpen-Momentary/5  "<InternalRequest>"
  Bus Selector/3 -> LeftDoor1ManualOpen-Momentary/3  "<InitVal>"
  Bus Selector/2 -> LeftDoor1ManualOpen-Momentary/2  "<Mode>"
  Bus Selector/1 -> LeftDoor1ManualOpen-Momentary/1  "<Value>"
  InputControl/1 -> Bus Selector/1

== system IOControls/ForEachVehicle/IOControls/Non-CabControl/InteriorDoorControls/LeftDoor2Coving ==
  note: States:
      | Closed
      | Open
  InputControl : Inport  OutDataTypeStr=Bus: BD_IOControls_In_InputControl
  Initialise : Inport  Port=2
  Bus Selector : BusSelector  OutputSignals=Value,Mode,InitVal,InternalRequest,Inhibit
  LeftDoor2Coving-Toggle : IOStateMachinesLib/Toggle  InitSource=internal  InitState=InitState  OffStateValue=OffStateValue  OnStateValue=OnStateValue
      settings: SourceProductName=IO State Machines
  InputState : Outport  VectorParamsAs1DForOutWhenUnconnected=off
  wires:
  Initialise/1 -> LeftDoor2Coving-Toggle/4
  LeftDoor2Coving-Toggle/1 -> InputState/1
  Bus Selector/5 -> LeftDoor2Coving-Toggle/6  "<Inhibit>"
  Bus Selector/4 -> LeftDoor2Coving-Toggle/5  "<InternalRequest>"
  Bus Selector/3 -> LeftDoor2Coving-Toggle/3  "<InitVal>"
  Bus Selector/2 -> LeftDoor2Coving-Toggle/2  "<Mode>"
  Bus Selector/1 -> LeftDoor2Coving-Toggle/1  "<Value>"
  InputControl/1 -> Bus Selector/1

== system IOControls/ForEachVehicle/IOControls/Non-CabControl/InteriorDoorControls/LeftDoor2DCUCB ==
  note: States:
      | Tripped
      | Set
  MCBControl : Inport  OutDataTypeStr=Bus: BD_IOControls_In_MCBControl
  Initialise : Inport  Port=2
  Bus Selector : BusSelector  OutputSignals=Value,Mode,InitVal,InternalRequest,Inhibit,TripRequest
  LeftDoor2DCUCB-MCB : IOStateMachinesLib/MCB  InitSource=internal  InitState=InitState  OffStateValue=OffStateValue  OnStateValue=OnStateValue
      settings: SourceProductName=IO State Machines
  InputState : Outport  VectorParamsAs1DForOutWhenUnconnected=off
  MCBTripState : Outport  Port=2  VectorParamsAs1DForOutWhenUnconnected=off
  wires:
  LeftDoor2DCUCB-MCB/2 -> MCBTripState/1
  Bus Selector/6 -> LeftDoor2DCUCB-MCB/7  "<TripRequest>"
  MCBControl/1 -> Bus Selector/1
  Bus Selector/1 -> LeftDoor2DCUCB-MCB/1  "<Value>"
  Bus Selector/2 -> LeftDoor2DCUCB-MCB/2  "<Mode>"
  Bus Selector/3 -> LeftDoor2DCUCB-MCB/3  "<InitVal>"
  Bus Selector/4 -> LeftDoor2DCUCB-MCB/5  "<InternalRequest>"
  Bus Selector/5 -> LeftDoor2DCUCB-MCB/6  "<Inhibit>"
  LeftDoor2DCUCB-MCB/1 -> InputState/1
  Initialise/1 -> LeftDoor2DCUCB-MCB/4

== system IOControls/ForEachVehicle/IOControls/Non-CabControl/InteriorDoorControls/LeftDoor2EED ==
  note: States:
      | Reset
      | Operated
  InputControl : Inport  OutDataTypeStr=Bus: BD_IOControls_In_InputControl
  Initialise : Inport  Port=2
  Bus Selector : BusSelector  OutputSignals=Value,Mode,InitVal,InternalRequest,Inhibit
  LeftDoor2EED-Momentary : IOStateMachinesLib/Momentary  InitSource=internal  InitState=InitState
      settings: SourceProductName=IO State Machines
  InputState : Outport  VectorParamsAs1DForOutWhenUnconnected=off
  wires:
  Initialise/1 -> LeftDoor2EED-Momentary/4
  LeftDoor2EED-Momentary/1 -> InputState/1
  Bus Selector/5 -> LeftDoor2EED-Momentary/6  "<Inhibit>"
  Bus Selector/4 -> LeftDoor2EED-Momentary/5  "<InternalRequest>"
  Bus Selector/3 -> LeftDoor2EED-Momentary/3  "<InitVal>"
  Bus Selector/2 -> LeftDoor2EED-Momentary/2  "<Mode>"
  Bus Selector/1 -> LeftDoor2EED-Momentary/1  "<Value>"
  InputControl/1 -> Bus Selector/1

== system IOControls/ForEachVehicle/IOControls/Non-CabControl/InteriorDoorControls/LeftDoor2Lockout ==
  note: States:
      | Unlocked
      | Locked
  InputControl : Inport  OutDataTypeStr=Bus: BD_IOControls_In_InputControl
  Initialise : Inport  Port=2
  Bus Selector : BusSelector  OutputSignals=Value,Mode,InitVal,InternalRequest,Inhibit
  LeftDoor2Lockout-Toggle : IOStateMachinesLib/Toggle  InitSource=internal  InitState=InitState  OffStateValue=OffStateValue  OnStateValue=OnStateValue
      settings: SourceProductName=IO State Machines
  InputState : Outport  VectorParamsAs1DForOutWhenUnconnected=off
  wires:
  Initialise/1 -> LeftDoor2Lockout-Toggle/4
  LeftDoor2Lockout-Toggle/1 -> InputState/1
  Bus Selector/5 -> LeftDoor2Lockout-Toggle/6  "<Inhibit>"
  Bus Selector/4 -> LeftDoor2Lockout-Toggle/5  "<InternalRequest>"
  Bus Selector/3 -> LeftDoor2Lockout-Toggle/3  "<InitVal>"
  Bus Selector/2 -> LeftDoor2Lockout-Toggle/2  "<Mode>"
  Bus Selector/1 -> LeftDoor2Lockout-Toggle/1  "<Value>"
  InputControl/1 -> Bus Selector/1
